simulink model "segmentCalcPos"  (R2019a)
settings: Solver=FixedStepAuto  StartTime=0  StopTime=inf  FixedStep=1e-3  MaxStep=1e-3  RelTol=1e-3
values from neighbouring files (symbols this model uses):
  apexVelocity = flippedVel(n)    [Untitled.m]    (also in calcSegments.m = apexData.velocity(n,2); testInit.m)
  course = [22.662224 22.6513857656 22.6409781601 22.6309993845 22.6214476087 22.6123209722 22.6036175847 22.5953355273 22.5874728529 22.5800275876 22.5729977309 22.5663812572 ... (23224 elements, 11612x2)]    [course_data_0_1m.mat]    (also in course_data_0_5m.mat = [22.662224 22.6123209722 22.5729977309 22.5440078299 22.5250; course_data_1m.mat = [22.516 22.544 22.607 22.702 22.826 22.981 23.17 23.398 23.6; importCourse.m = table2array(course))
  currentDistance = (flippedLocs(n) - 1) * init.ptDistance    [Untitled.m]    (also in calcSegments.m = (apexData.locs(n,1) - 1) * init.ptDistance; testInit.m)
  flippedCourse = flip(course)    [Untitled.m]    (also in calcSegments.m; testInit.m)
  init =     [course_data_0_1m.mat]
  stoppingDistance = (flippedLocs(n+1) - 1) * init.ptDistance    [Untitled.m]    (also in calcSegments.m = (apexData.locs(n+1,1) - 1) * init.ptDistance; testInit.m)
  TrackLength = 1161.1    [course_data_0_1m.mat]    (also in course_data_0_5m.mat = 1161; course_data_1m.mat = 1161; sortingPoints.m = (length(courseSorted)-1) * evalin('base', 'init.ptDistance'))
libraries: simulink x1
settings Model: Creator=Frieder Uerlings  LastModifiedBy=Frieder Uerlings
settings SolverCC: ZeroCrossControl=DisableAll  AlgebraicLoopSolver=LineSearch

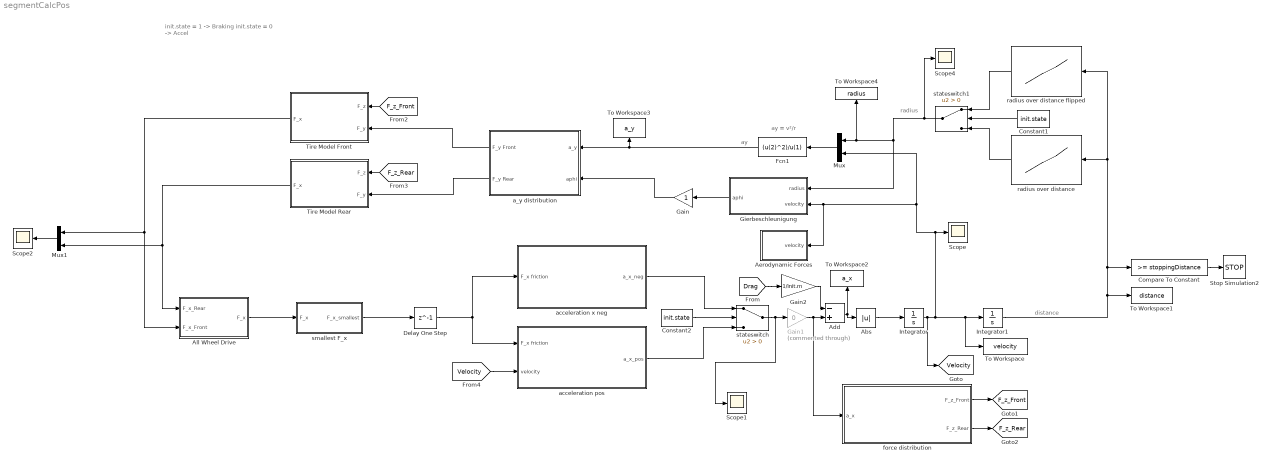
== system segmentCalcPos ==
  note: ay = v²/r
  note: init.state = 1 -> Braking
      | init.state = 0 -> Accel
  note: radius
  note: distance
  note: ay
  Abs : Abs
  Add : Sum  Inputs=-+
  Aerodynamic Forces : Subsystem
  All Wheel Drive : Subsystem
  Compare To Constant : simulink/Logic and Bit Operations/Compare To Constant  relop=>=  const=stoppingDistance  OutDataTypeStr=boolean
  Constant1 : Constant  Value=init.state
  Constant2 : Constant  Value=init.state
  Delay One Step : Delay  DelayLength=1  InitialCondition=0  InputProcessing=Columns as channels (frame based)
  Fcn1 : Fcn  Expr=(u(2)^2)/u(1)
  Gain : Gain
  Gain1 : Gain  Commented=through  Gain=0
  Gain2 : Gain  Gain=1/init.m
  Gierbeschleunigung : Subsystem
  Integrator : Integrator  InitialCondition=apexVelocity
  Integrator1 : Integrator  InitialCondition=currentDistance
  Mux : Mux  Inputs=2
  Mux1 : Mux  Inputs=2
  Scope{,1..2,4} (4 alike) : Scope
  Stop Simulation2 : Stop
  Tire Model Front : Subsystem
  Tire Model Rear : Subsystem
  To Workspace : ToWorkspace  VariableName=velocity  SampleTime=-1
  To Workspace1 : ToWorkspace  VariableName=distance  SampleTime=-1
  To Workspace2 : ToWorkspace  VariableName=a_x  SampleTime=-1
  To Workspace3 : ToWorkspace  VariableName=a_y  SampleTime=-1
  To Workspace4 : ToWorkspace  VariableName=radius  SampleTime=-1
  a_y distribution : Subsystem
  "acceleration pos " : Subsystem
  acceleration x neg : Subsystem
  force distribution : Subsystem
  radius over distance : Lookup_n-D  NumberOfTableDimensions=1  BreakpointsForDimension1=[0:init.ptDistance:TrackLength]  Table=course(:,3)  InternalRulePriority=Speed  RndMeth=Simplest  InputSameDT=on
  radius over distance flipped : Lookup_n-D  NumberOfTableDimensions=1  BreakpointsForDimension1=[0:init.ptDistance:TrackLength]  Table=flippedCourse(:,3)  InternalRulePriority=Speed  RndMeth=Simplest  InputSameDT=on
  smallest F_x : Subsystem
  stateswitch : Switch  Criteria=u2 > Threshold
  stateswitch1 : Switch  Criteria=u2 > Threshold
  tag scope: F_z_Front=global, F_z_Rear=global, Velocity=global
  wires:
  Mux/1 -> Fcn1/1
  Compare To Constant/1 -> Stop Simulation2/1
  Integrator/1 -> [Velocity], To Workspace/1, Integrator1/1, Aerodynamic Forces/1(velocity), Gierbeschleunigung/2("velocity "), Mux/2, Scope/1
  stateswitch/1 -> Scope1/1, Gain1/1
  Fcn1/1 -> a_y distribution/1("a_y "), To Workspace3/1
  Integrator1/1 -> radius over distance flipped/1, radius over distance/1, Compare To Constant/1, To Workspace1/1
  a_y distribution/1("F_y Front ") -> Tire Model Front/2(F_y)
  force distribution/1(F_z_Front) -> [F_z_Front]
  force distribution/2("F_z_Rear ") -> [F_z_Rear]
  [F_z_Front] -> Tire Model Front/1(F_z)
  a_y distribution/2("F_y Rear ") -> Tire Model Rear/2(F_y)
  [F_z_Rear] -> Tire Model Rear/1(F_z)
  Gierbeschleunigung/1(aphi) -> Gain/1
  Delay One Step/1 -> "acceleration pos "/1(F_x friction), acceleration x neg/1(F_x friction)
  Constant2/1 -> stateswitch/2
  acceleration x neg/1("a_x_neg ") -> stateswitch/1
  "acceleration pos "/1("a_x_pos ") -> stateswitch/3
  Tire Model Front/1(F_x) -> Mux1/1, All Wheel Drive/2(F_x_Front)
  Tire Model Rear/1(F_x) -> All Wheel Drive/1(F_x_Rear), Mux1/2
  radius over distance flipped/1 -> stateswitch1/1
  radius over distance/1 -> stateswitch1/3
  stateswitch1/1 -> Scope4/1, Gierbeschleunigung/1(radius), To Workspace4/1, Mux/1
  [Velocity] -> "acceleration pos "/2(velocity)
  Constant1/1 -> stateswitch1/2
  Abs/1 -> Integrator/1
  All Wheel Drive/1(F_x) -> smallest F_x/1("F_x ")
  Gain/1 -> a_y distribution/2("aphi ")
  Mux1/1 -> Scope2/1
  Gain1/1 -> Add/2, force distribution/1("a_x ")
  smallest F_x/1(F_x_smallest) -> Delay One Step/1
  Add/1 -> To Workspace2/1, Abs/1
  [Drag] -> Gain2/1
  Gain2/1 -> Add/1

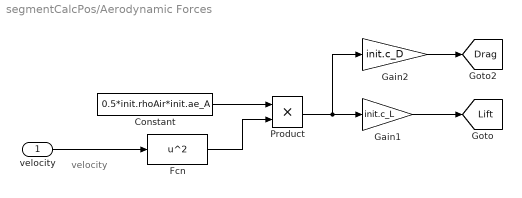
== system segmentCalcPos/Aerodynamic Forces ==
  note: velocity
  velocity : Inport
  Constant : Constant  Value=0.5*init.rhoAir*init.ae_A
  Fcn : Fcn  Expr=u^2
  Gain1 : Gain  Gain=init.c_L
  Gain2 : Gain  Gain=init.c_D
  Product : Product
  tag scope: Drag=global, Lift=global
  wires:
  Fcn/1 -> Product/2
  Constant/1 -> Product/1
  Product/1 -> Gain2/1, Gain1/1
  Gain1/1 -> [Lift]
  velocity/1 -> Fcn/1
  Gain2/1 -> [Drag]

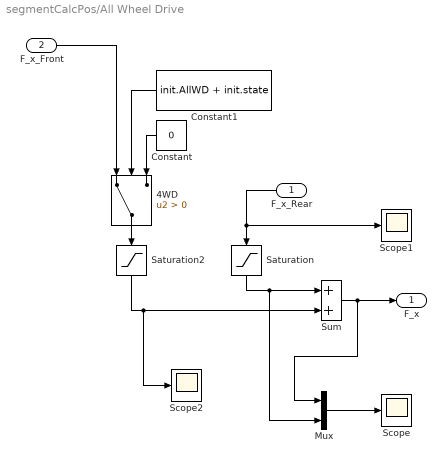
== system segmentCalcPos/All Wheel Drive ==
  F_x_Rear : Inport
  F_x_Front : Inport  Port=2
  4WD : Switch  Criteria=u2 > Threshold
  Constant : Constant  Value=0
  Constant1 : Constant  Value=init.AllWD + init.state
  Mux : Mux  Inputs=2
  Saturation : Saturate  UpperLimit=inf  LowerLimit=0
  Saturation2 : Saturate  UpperLimit=inf  LowerLimit=0
  Scope : Scope
  Scope1 : Scope
  Scope2 : Scope
  Sum : Sum
  F_x : Outport
  wires:
  Constant1/1 -> 4WD/2
  F_x_Rear/1 -> Scope1/1, Saturation/1
  4WD/1 -> Saturation2/1
  Constant/1 -> 4WD/3
  F_x_Front/1 -> 4WD/1
  Saturation/1 -> Mux/2, Sum/1
  Saturation2/1 -> Scope2/1, Sum/2
  Sum/1 -> Mux/1, F_x/1
  Mux/1 -> Scope/1

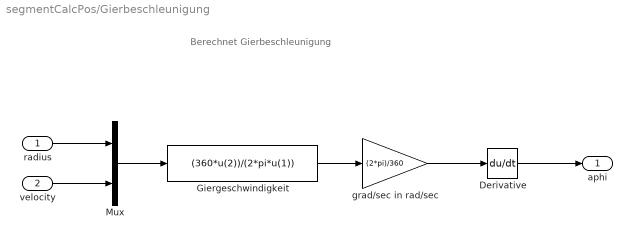
== system segmentCalcPos/Gierbeschleunigung ==
  note: Berechnet Gierbeschleunigung
  radius : Inport
  "velocity " : Inport  Port=2
  Derivative : Derivative
  Giergeschwindigkeit : Fcn  Expr=(360*u(2))/(2*pi*u(1))
  Mux : Mux  Inputs=2
  grad/sec in rad/sec : Gain  Gain=(2*pi)/360
  aphi : Outport
  wires:
  radius/1 -> Mux/1
  "velocity "/1 -> Mux/2
  Mux/1 -> Giergeschwindigkeit/1
  Giergeschwindigkeit/1 -> grad/sec in rad/sec/1
  grad/sec in rad/sec/1 -> Derivative/1
  Derivative/1 -> aphi/1

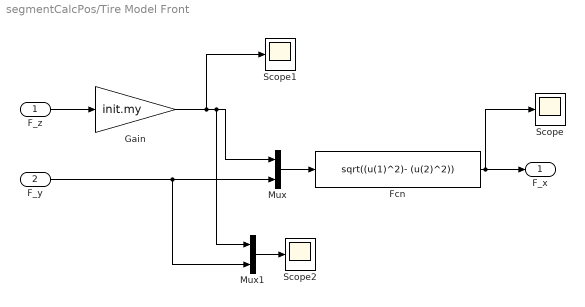
== system segmentCalcPos/Tire Model Front ==
  F_z : Inport
  F_y : Inport  Port=2
  Fcn : Fcn  Expr=sqrt((u(1)^2)- (u(2)^2))
  Gain : Gain  Gain=init.my
  Mux : Mux  Inputs=2
  Mux1 : Mux  Inputs=2
  Scope : Scope
  Scope1 : Scope
  Scope2 : Scope
  F_x : Outport
  wires:
  F_z/1 -> Gain/1
  Mux/1 -> Fcn/1
  F_y/1 -> Mux1/2, Mux/2
  Fcn/1 -> Scope/1, F_x/1
  Gain/1 -> Scope1/1, Mux1/1, Mux/1
  Mux1/1 -> Scope2/1

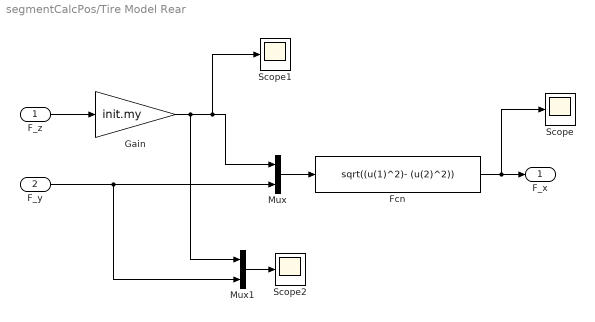
== system segmentCalcPos/Tire Model Rear ==
  F_z : Inport
  F_y : Inport  Port=2
  Fcn : Fcn  Expr=sqrt((u(1)^2)- (u(2)^2))
  Gain : Gain  Gain=init.my
  Mux : Mux  Inputs=2
  Mux1 : Mux  Inputs=2
  Scope : Scope
  Scope1 : Scope
  Scope2 : Scope
  F_x : Outport
  wires:
  F_y/1 -> Mux1/2, Mux/2
  Gain/1 -> Mux1/1, Scope1/1, Mux/1
  Mux/1 -> Fcn/1
  Fcn/1 -> Scope/1, F_x/1
  F_z/1 -> Gain/1
  Mux1/1 -> Scope2/1

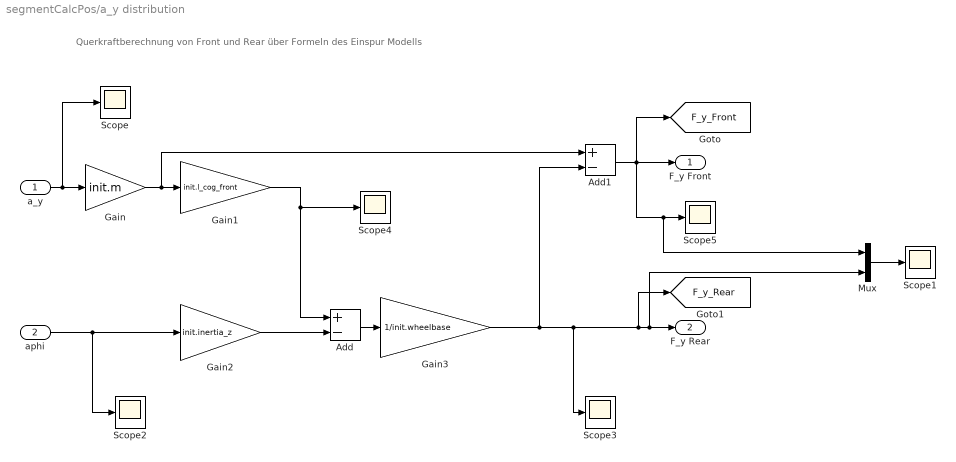
== system segmentCalcPos/a_y distribution ==
  note: Querkraftberechnung von Front und Rear über Formeln des Einspur Modells
  "a_y " : Inport
  "aphi " : Inport  Port=2
  Add : Sum  Inputs=+-
  Add1 : Sum  Inputs=+-
  Gain : Gain  Gain=init.m
  Gain1 : Gain  Gain=init.l_cog_front
  Gain2 : Gain  Gain=init.inertia_z
  Gain3 : Gain  Gain=1/init.wheelbase
  Mux : Mux  Inputs=2
  Scope{,1..5} (6 alike) : Scope
  "F_y Front " : Outport
  "F_y Rear " : Outport  Port=2
  tag scope: F_y_Front=global, F_y_Rear=global
  wires:
  "a_y "/1 -> Scope/1, Gain/1
  Gain/1 -> Add1/1, Gain1/1
  Gain1/1 -> Scope4/1, Add/1
  Gain2/1 -> Add/2
  "aphi "/1 -> Scope2/1, Gain2/1
  Add/1 -> Gain3/1
  Gain3/1 -> Add1/2, Scope3/1, [F_y_Rear], Mux/2, "F_y Rear "/1
  Add1/1 -> [F_y_Front], Mux/1, Scope5/1, "F_y Front "/1
  Mux/1 -> Scope1/1

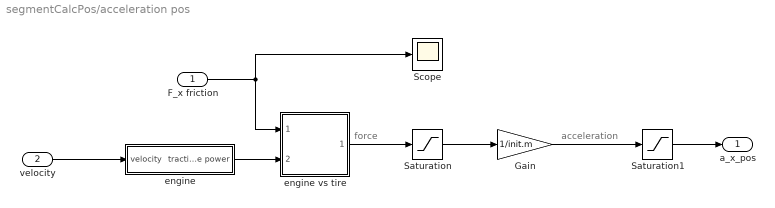
== system segmentCalcPos/acceleration pos  ==
  note: force
  note: acceleration
  F_x friction : Inport
  velocity : Inport  Port=2
  Gain : Gain  Gain=1/init.m
  Saturation : Saturate  UpperLimit=inf  LowerLimit=0
  Saturation1 : Saturate  UpperLimit=inf  LowerLimit=0  ZeroCross=off
  Scope : Scope
  engine : Subsystem
  engine vs tire : Subsystem
  "a_x_pos " : Outport
  wires:
  Gain/1 -> Saturation1/1
  engine vs tire/1(acc force) -> Saturation/1
  engine/1(tractive power) -> engine vs tire/2(tractive power)
  F_x friction/1 -> engine vs tire/1("a_x friction "), Scope/1
  velocity/1 -> engine/1(velocity)
  Saturation/1 -> Gain/1
  Saturation1/1 -> "a_x_pos "/1

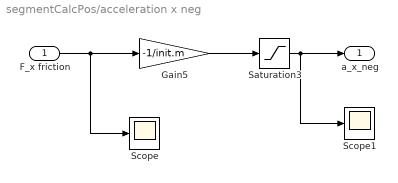
== system segmentCalcPos/acceleration x neg ==
  F_x friction : Inport
  Gain5 : Gain  Gain=-1/init.m
  Saturation3 : Saturate  UpperLimit=0  LowerLimit=-inf  ZeroCross=off
  Scope : Scope
  Scope1 : Scope
  "a_x_neg " : Outport
  wires:
  F_x friction/1 -> Gain5/1, Scope/1
  Gain5/1 -> Saturation3/1
  Saturation3/1 -> Scope1/1, "a_x_neg "/1

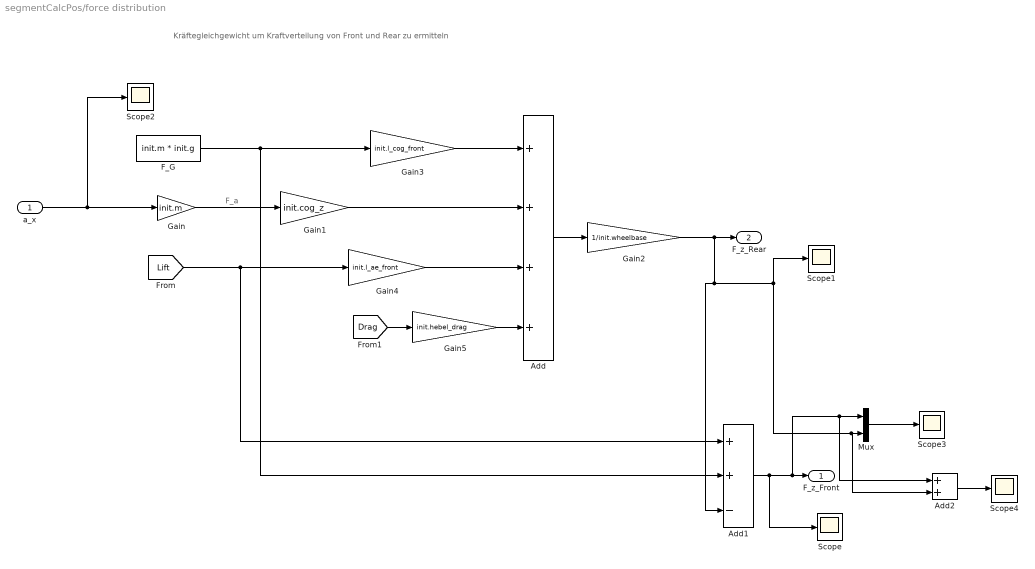
== system segmentCalcPos/force distribution ==
  note: Kräftegleichgewicht um Kraftverteilung von Front und Rear zu ermitteln
  note: F_a
  "a_x " : Inport
  Add : Sum  Inputs=++++
  Add1 : Sum  Inputs=++-
  Add2 : Sum
  "F_G " : Constant  Value=init.m * init.g
  Gain : Gain  Gain=init.m
  Gain1 : Gain  Gain=init.cog_z
  Gain2 : Gain  Gain=1/init.wheelbase
  Gain3 : Gain  Gain=init.l_cog_front
  Gain4 : Gain  Gain=init.l_ae_front
  Gain5 : Gain  Gain=init.hebel_drag
  Mux : Mux  Inputs=2
  Scope{,1..4} (5 alike) : Scope
  F_z_Front : Outport
  "F_z_Rear " : Outport  Port=2
  wires:
  "F_G "/1 -> Add1/2, Gain3/1
  Gain3/1 -> Add/1
  Gain/1 -> Gain1/1
  [Lift] -> Gain4/1, Add1/1
  Gain1/1 -> Add/2
  Gain4/1 -> Add/3
  Add/1 -> Gain2/1
  Gain2/1 -> Add1/3, Scope1/1, Add2/2, Mux/2, "F_z_Rear "/1
  Add1/1 -> Scope/1, Add2/1, Mux/1, F_z_Front/1
  Mux/1 -> Scope3/1
  Add2/1 -> Scope4/1
  "a_x "/1 -> Gain/1, Scope2/1
  Gain5/1 -> Add/4
  [Drag] -> Gain5/1

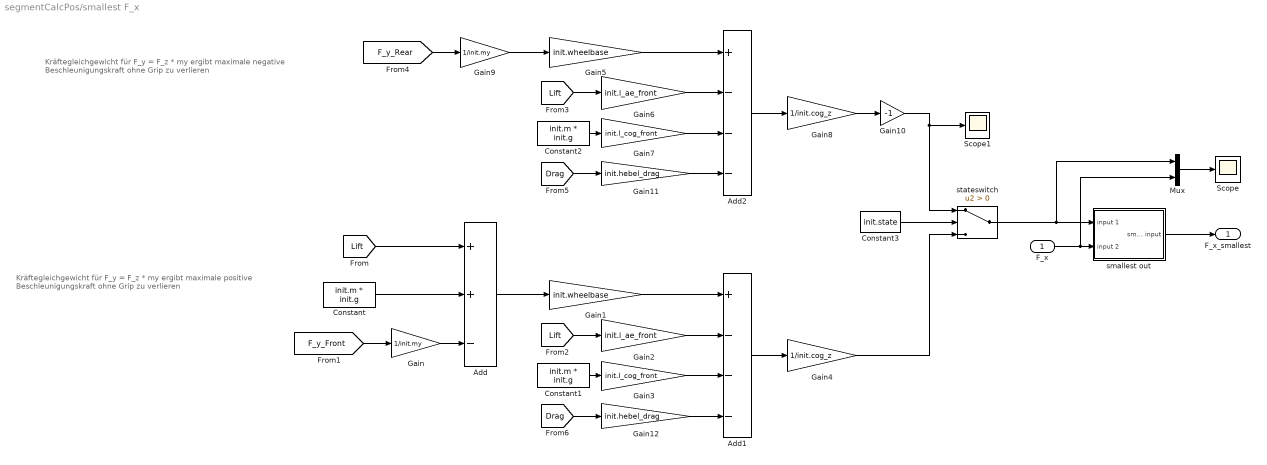
== system segmentCalcPos/smallest F_x ==
  note: Kräftegleichgewicht für F_y = F_z * my
      | ergibt maximale positive Beschleunigungskraft
      | ohne Grip zu verlieren
  note: Kräftegleichgewicht für F_y = F_z * my
      | ergibt maximale negative Beschleunigungskraft
      | ohne Grip zu verlieren
  "F_x " : Inport
  Add : Sum  Inputs=++-
  Add1 : Sum  Inputs=+---
  Add2 : Sum  Inputs=+---
  Constant : Constant  Value=init.m * init.g
  Constant1 : Constant  Value=init.m * init.g
  Constant2 : Constant  Value=init.m * init.g
  Constant3 : Constant  Value=init.state
  Gain : Gain  Gain=1/init.my
  Gain1 : Gain  Gain=init.wheelbase
  Gain10 : Gain  Gain=-1
  Gain11 : Gain  Gain=init.hebel_drag
  Gain12 : Gain  Gain=init.hebel_drag
  Gain2 : Gain  Gain=init.l_ae_front
  Gain3 : Gain  Gain=init.l_cog_front
  Gain4 : Gain  Gain=1/init.cog_z
  Gain5 : Gain  Gain=init.wheelbase
  Gain6 : Gain  Gain=init.l_ae_front
  Gain7 : Gain  Gain=init.l_cog_front
  Gain8 : Gain  Gain=1/init.cog_z
  Gain9 : Gain  Gain=1/init.my
  Mux : Mux  Inputs=2
  Scope : Scope
  Scope1 : Scope
  smallest out : Subsystem
  stateswitch : Switch  Criteria=u2 > Threshold
  F_x_smallest : Outport
  wires:
  [Lift] -> Add/1
  Constant/1 -> Add/2
  [F_y_Front] -> Gain/1
  Gain/1 -> Add/3
  Add/1 -> Gain1/1
  Gain1/1 -> Add1/1
  [Lift] -> Gain2/1
  Gain2/1 -> Add1/2
  Constant1/1 -> Gain3/1
  Gain3/1 -> Add1/3
  Add1/1 -> Gain4/1
  "F_x "/1 -> Mux/2, smallest out/2(input 2)
  smallest out/1(smallest input) -> F_x_smallest/1
  Add2/1 -> Gain8/1
  Gain7/1 -> Add2/3
  Constant2/1 -> Gain7/1
  Gain6/1 -> Add2/2
  [Lift] -> Gain6/1
  Gain5/1 -> Add2/1
  [F_y_Rear] -> Gain9/1
  Gain9/1 -> Gain5/1
  Constant3/1 -> stateswitch/2
  Gain8/1 -> Gain10/1
  Gain4/1 -> stateswitch/3
  stateswitch/1 -> Mux/1, smallest out/1("input 1 ")
  Mux/1 -> Scope/1
  Gain10/1 -> Scope1/1, stateswitch/1
  [Drag] -> Gain11/1
  Gain11/1 -> Add2/4
  [Drag] -> Gain12/1
  Gain12/1 -> Add1/4

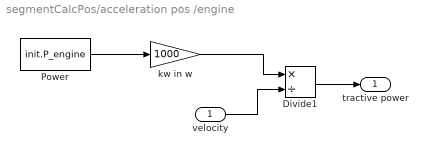
== system segmentCalcPos/acceleration pos /engine ==
  velocity : Inport
  Divide1 : Product  Inputs=*/
  "Power " : Constant  Value=init.P_engine
  "kw in w " : Gain  Gain=1000
  tractive power : Outport
  wires:
  "Power "/1 -> "kw in w "/1
  "kw in w "/1 -> Divide1/1
  Divide1/1 -> tractive power/1
  velocity/1 -> Divide1/2

== system segmentCalcPos/acceleration pos /engine vs tire ==
  note: max force
  note: max friction force
  "a_x friction " : Inport
  tractive power : Inport  Port=2
  Relational Operator : RelationalOperator  Operator=<=  OutDataTypeStr=boolean  RndMeth=Simplest
  Switch : Switch  Criteria=u2 > Threshold
  acc force : Outport
  wires:
  tractive power/1 -> Relational Operator/2, Switch/3
  "a_x friction "/1 -> Relational Operator/1, Switch/1
  Switch/1 -> acc force/1
  Relational Operator/1 -> Switch/2

== system segmentCalcPos/smallest F_x/smallest out ==
  "input 1 " : Inport
  input 2 : Inport  Port=2
  Relational Operator : RelationalOperator  Operator=<=  OutDataTypeStr=boolean  RndMeth=Simplest
  Switch : Switch  Criteria=u2 > Threshold
  smallest input : Outport
  wires:
  input 2/1 -> Relational Operator/2, Switch/3
  "input 1 "/1 -> Relational Operator/1, Switch/1
  Switch/1 -> smallest input/1
  Relational Operator/1 -> Switch/2
